simulink model "simple_streaming_txrx"  (Simulink 6.6)
settings: Solver=ode45  StartTime=0.0  StopTime=inf  RelTol=1e-3
InitFcn:
  | simple_streaming_init
StartFcn:
  | simple_streaming_init
undefined symbols (not defined in the file): dmf, gcbh, get, modConstellation_qam16, modConstellation_qam64, modConstellation_qpsk, rcosfir, symbolRomLen, txLSFR_initValues, txLSFR_polynomials, viqAvgLen, xlBlockLoadCallback, xlGetSimulinkPeriod
libraries: xbsIndex_r4 x506, commchan3 x2, commsink2 x1
(part 1 of 5)
settings Model: Creator=chunter  LastModifiedBy=chunter

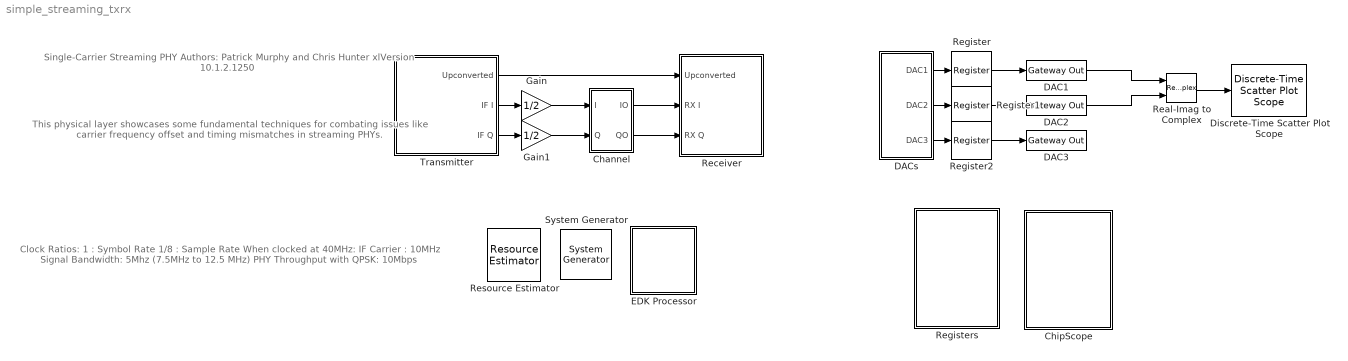
== system simple_streaming_txrx ==
  note: Single-Carrier Streaming PHY
      | Authors: Patrick Murphy and Chris Hunter
      | xlVersion 10.1.2.1250
  note: This physical layer showcases some fundamental
      | techniques for combating issues like carrier frequency
      | offset and timing mismatches in streaming PHYs.
  note: Clock Ratios:
      | 1 : Symbol Rate
      | 1/8 : Sample Rate
      |
      | When clocked at 40MHz:
      | IF Carrier : 10MHz
      | Signal Bandwidth: 5Mhz (7.5MHz to 12.5 MHz)
      | PHY Throughput with QPSK: 10Mbps
  " System Generator" : xbsIndex_r4/ System Generator  Tag=genX  SystemSampleTime=-1  xilinxfamily=virtex2p  part=xc2vp70  speed=-6  package=ff1517  synthesis_tool=XST  clock_wrapper=Clock Enables  directory=./netlist  testbench=off  simulink_period=1/8  sysclk_period=10  dcm_input_clock_period=100  incr_netlist=off  trim_vbits=Everywhere in SubSystem  dbl_ovrd=According to Block Masks  core_generation=According to Block Masks  run_coregen=off  deprecated_control=off  eval_field=0  block_type=sysgen
      settings: block_version=10.1.2
  Channel : Subsystem
  ChipScope : Subsystem
  DAC1 : xbsIndex_r4/Gateway Out  hdl_port=on  timing_constraint=None  locs_specified=off  LOCs={}  block_type=gatewayout
      settings: infoedit="Gateway out block.  Converts Xilinx fixed point inputs into ouputs of type Simulink integer, double, or fixed point.<P><P>Hardware notes:  In hardware these blocks become top level output ports or are discarded, depending on how they are configured."  xl_area=[0 0 0 0 14 0 0]  block_version=10.1
  DAC2 : xbsIndex_r4/Gateway Out  hdl_port=on  timing_constraint=None  locs_specified=off  LOCs={}  block_type=gatewayout
      settings: infoedit="Gateway out block.  Converts Xilinx fixed point inputs into ouputs of type Simulink integer, double, or fixed point.<P><P>Hardware notes:  In hardware these blocks become top level output ports or are discarded, depending on how they are configured."  xl_area=[0 0 0 0 14 0 0]  block_version=10.1
  DAC3 : xbsIndex_r4/Gateway Out  hdl_port=on  timing_constraint=None  locs_specified=off  LOCs={}  block_type=gatewayout
      settings: infoedit="Gateway out block.  Converts Xilinx fixed point inputs into ouputs of type Simulink integer, double, or fixed point.<P><P>Hardware notes:  In hardware these blocks become top level output ports or are discarded, depending on how they are configured."  xl_area=[0 0 0 0 14 0 0]  block_version=10.1
  DACs : Subsystem
  Discrete-Time Scatter Plot Scope : commsink2/Discrete-Time Scatter Plot Scope  Tag=ScatterPlot  SystemSampleTime=-1  sampPerSymb=1  offsetEye=0  numTraces=40  numNewFrames=10  LineMarkers=.  LineColors=b  fading=on  render=on  AxisGrid=on  xMin=-3.3  xMax=3.315  yMin=-3.3  yMax=3.315  inphaseLabel=In-phase Amplitude  quadratureLabel=Quadrature Amplitude  openScopeAtSimStart=on  FrameNumber=off  FigPos=get(0,'defaultfigureposition');  figTitle=Scatter Plot  numLinesMax=8  block_type_=scatter
  EDK Processor : Subsystem  LoadFcn=xlBlockLoadCallback(gcbh);  mask(Xilinx EDK Processor Block){mode=EDK pcore generation, xmp=, MemVisToProc=<qt bgcolor="#FFFFFF"><div><img src="C:\Xilinx\10.1\DSP_Tools\common\bin\..\..\sysgen\data\images\registerminus.gif"> &lt;&lt;cfoEnable&gt;&gt;<br> <img src="C:\Xilinx\10.1\DSP_Tools\common\bin\..\..\sysgen\data\images\parameters.gif"> Type : UFix_1_0<br> <img src="C:\Xilinx\10.1\DSP_Tools\common\bin\..\..\sysgen\data\images\parameters.gif"> Addr : 0x80000800<br></div><div><img src="C:\Xilinx\10.1\DSP_Tools\common\bin\..\..\sysgen\data\images\registerplus.gif"> &lt;&lt;cfoK&gt;&gt;<br></div><div><img src="C:\Xilinx\10.1\DSP_Tools\common\bin\..\..\sysgen\data\images\registerplus.gif"> &lt;&lt;cfoKI&gt;&gt;<br></div><div><img src="C:\Xilinx\10.1\DSP_Tools\common\bin\..\..\sysgen\data\images\registerplus.gif"> &lt;&lt;cfoKP&gt;&gt;<br></div><div><img src="C:\Xilinx\10.1\DSP_Tools\common\bin\..\..\sysgen\data\images\registerplus.gif"> &lt;&lt;cfoReset&gt;&gt;<br></div><div><img src="C:\Xilinx\10.1\DSP_Tools\common\bin\..\..\sysgen\data\images\registerplus.gif"> &lt;&lt;dac1Sel&gt;&gt;<br></div><div><img src="C:\Xilinx\10.1\DSP_Tools\common\bin\..\..\sysgen\data\images\registerplus.gif"> &lt;&lt;dac2Sel&gt;&gt;<br></div><div><img src="C:\Xilinx\10.1\DSP_Tools\common\bin\..\..\sysgen\data\images\registerplus.gif"> &lt;&lt;dac3Sel&gt;&gt;<br></div><div><img src="C:\Xilinx\10.1\DSP_Tools\common\bin\..\..\sysgen\data\images\registerplus.gif"> &lt;&lt;downConv&gt;&gt;<br></div><div><img src="C:\Xilinx\10.1\DSP_Tools\common\bin\..\..\sysgen\data\images\registerplus.gif"> &lt;&lt;initialDelay&gt;&gt;<br></div><div><img src="C:\Xilinx\10.1\DSP_Tools\common\bin\..\..\sysgen\data\images\registerminus.gif"> &lt;&lt;otrBenefit&gt;&gt;<br> <img src="C:\Xilinx\10.1\DSP_Tools\common\bin\..\..\sysgen\data\images\parameters.gif"> Type : UFix_32_0<br> <img src="C:\Xilinx\10.1\DSP_Tools\common\bin\..\..\sysgen\data\images\parameters.gif"> Addr : 0x80000828<br></div><div><img src="C:\Xilinx\10.1\DSP_Tools\common\bin\..\..\sysgen\data\images\registerplus.gif"> &lt;&lt;otrCost&gt;&gt;<br></div><div><img src="C:\Xilinx\10.1\DSP_Tools\common\bin\..\..\sysgen\data\images\registerplus.gif"> &lt;&lt;rxInputSel&gt;&gt;<br></div><div><img src="C:\Xilinx\10.1\DSP_Tools\common\bin\..\..\sysgen\data\images\registerplus.gif"> &lt;&lt;timingK&gt;&gt;<br></div><div><img src="C:\Xilinx\10.1\DSP_Tools\common\bin\..\..\sysgen\data\images\registerplus.gif"> &lt;&lt;timingKI&gt;&gt;<br></div><div><img src="C:\Xilinx\10.1\DSP_Tools\common\bin\..\..\sysgen\data\images\registerplus.gif"> &lt;&lt;timingKP&gt;&gt;<br></div><div><img src="C:\Xilinx\10.1\DSP_Tools\common\bin\..\..\sysgen\data\images\registerplus.gif"> &lt;&lt;timingReset&gt;&gt;<br></div><div><img src="C:\Xilinx\10.1\DSP_Tools\common\bin\..\..\sysgen\data\images\registerplus.gif"> &lt;&lt;txModSel&gt;&gt;<br></div><div><img src="C:\Xilinx\10.1\DSP_Tools\common\bin\..\..\sysgen\data\images\registerminus.gif"> &lt;&lt;upConv&gt;&gt;<br> <img src="C:\Xilinx\10.1\DSP_Tools\common\bin\..\..\sysgen\data\images\parameters.gif"> Type : UFix_32_0<br> <img src="C:\Xilinx\10.1\DSP_Tools\common\bin\..\..\sysgen\data\images\parameters.gif"> Addr : 0x80000848<br></div><div><img src="C:\Xilinx\10.1\DSP_Tools\common\bin\..\..\sysgen\data\images\registerminus.gif"> &lt;&lt;otr&gt;&gt;<br> <img src="C:\Xilinx\10.1\DSP_Tools\common\bin\..\..\sysgen\data\images\parameters.gif"> Type : UFix_32_0<br> <img src="C:\Xilinx\10.1\DSP_Tools\common\bin\..\..\sysgen\data\images\parameters.gif"> Addr : 0x80000850<br></div><div><img src="C:\Xilinx\10.1\DSP_Tools\common\bin\..\..\sysgen\data\images\registerminus.gif"> &lt;&lt;rssi&gt;&gt;<br> <img src="C:\Xilinx\10.1\DSP_Tools\common\bin\..\..\sysgen\data\images\parameters.gif"> Type : UFix_32_0<br> <img src="C:\Xilinx\10.1\DSP_Tools\common\bin\..\..\sysgen\data\images\parameters.gif"> Addr : 0x80000854<br></div><div><img src="C:\Xilinx\10.1\DSP_Tools\common\bin\..\..\sysgen\data\images\registerplus.gif"> &lt;&lt;viq&gt;&gt;<br></div><div><img src="C:\Xilinx\10.1\DSP_Tools\common\bin\..\..\sysgen\data\images\registerplus.gif"> &lt;&lt;viqReset&gt;&gt;<br></div></qt>, AvailableMemories=<empty>, portInterfaceTable={'exposed'=>[],'portdir'=>[],'portname'=>[],'shortname'=>[]}, bus_type_sgadvanced=, bus_type=PLB, baseaddr=0x80000000, baseaddr_lock_sgadvanced=, baseaddr_lock=off, dual_clock_sgadvanced=, dual_clock=off, ucf_file=, inheritDeviceType_sgadvanced=, inheritDeviceType=off, clock_name=plb, internalPortList={}, resetPolarity=0, memxtable={'mlist'=>['simple_streaming_txrx/Registers/From Register16','simple_streaming_txrx/Registers/From Register12','simple_streaming_txrx/Registers/From Register13','simple_streaming_txrx/Registers/From Register14','simple_streaming_txrx/Registers/From Register11','simple_streaming_txrx/Registers/From Register','simple_streaming_txrx/Registers/From Register1','simple_streaming_txrx/Registers/From Register4','simple_streaming_txrx/Registers/From Register5','simple_streaming_txrx/Registers/From Register15','simple_streaming_txrx/Registers/From Register17','simple_streaming_txrx/Registers/From Register18','simple_streaming_txrx/Registers/From Register6','simple_streaming_txrx/Registers/From Register7','simple_streaming_txrx/Registers/From Register9','simple_streaming_txrx/Registers/From Register8','simple_streaming_txrx/Registers/From Register10','simple_streaming_txrx/Registers/From Register2','simple_streaming_txrx/Registers/From Register3','simple_streaming_txrx/Registers/To Register2','simple_streaming_txrx/Registers/To Register1','simple_streaming_txrx/Registers/To Register','simple_streaming_txrx/Registers/From Register19'],'mlname'=>['\'cfoEnable\'','\'cfoK\'','\'cfoKI\'','\'cfoKP\'','\'cfoReset\'','\'dac1Sel\'','\'dac2Sel\'','\'dac3Sel\'','\'downConv\'','\'initialDelay\'','\'otrBenefit\'','\'otrCost\'','\'rxInputSel\'','\'timingK\'','\'timingKI\'','\'timingKP\'','\'timingReset\'','\'txModSel\'','\'upConv\'','\'otr\'','\'rssi\'','\'viq\'','\'viqReset\''],'mlstate'=>[1.0000000000000000,0.00000000000000000,0.00000000000000000,0.00000000000000000,0.00000000000000000,0.00000000000000000,0.00000000000000000,0.00000000000000000,0.00000000000000000,0.00000000000000000,1.0000000000000000,0.00000000000000000,0.00000000000000000,0.00000000000000000,0.00000000000000000,0.00000000000000000,0.00000000000000000,0.00000000000000000,1.0000000000000000,1.0000000000000000,1.0000000000000000,0.00000000000000000,0.00000000000000000]}, procinfo={'xmliface'=>'Xilinx//microblaze//iface.xml'}, fslifaceports=[0,0], memmapdirty=off, blockname=, xpsintstyle=default, proc=, has_advanced_control=0, sggui_pos=20,20,383,441, block_type=edkprocessor, block_version=2.4, sg_icon_stat=62,64,-1,-1,white,blue,0,07734,right, sg_mask_display=|, sg_list_contents={'table'=>{'AvailableMemories'=>'popup(<empty>)','userSelections'=>{'AvailableMemories'=>'<empty>'}}}, sg_blockgui_xml=}
      mask sg_mask_display=|
      | fprintf('','COMMENT: begin icon graphics');
      | patch([0 62 62 0 ],[0 0 64 64 ],[0.77 0.82 0.91]);
      | patch([14 4 19 4 14 30 34 38 56 42 29 19 33 19 29 42 56 38 34 30 14 ],[8 18 33 48 58 58 54 58 58 44 57 47 33 19 9 22 8 8 12 8 8 ],[0.98 0.96 0.92]);
      | plot([0 62 62 0 0 ],[0 0 64 64 0 ]);
      | fprintf('','COMMENT: end icon graphics');
      | fprintf('','COMMENT: begin icon text');
      | fprintf('','COMMENT: end icon text');
      mask prompts: mode "Configure Processor for"; xmp "EDK Project"; MemVisToProc ""; AvailableMemories "Available Memories"; portInterfaceTable ""; bus_type_sgadvanced ""; bus_type "Bus Type"; baseaddr "Base Address"; baseaddr_lock_sgadvanced ""; baseaddr_lock "Lock"; dual_clock_sgadvanced ""; dual_clock "Dual Clocks"; ucf_file "Constraint file"; inheritDeviceType_sgadvanced ""; inheritDeviceType "Inherit Device Type"; clock_name ""; internalPortList ""; resetPolarity ""; memxtable ""; procinfo ""; fslifaceports ""; memmapdirty ""; blockname ""; xpsintstyle ""; proc ""; has_advanced_control ""; sggui_pos ""; block_type ""; block_version ""; sg_icon_stat ""; sg_mask_display ""; sg_list_contents ""; sg_blockgui_xml ""
      mask help: Xilinx EDK Processor
      mask init:
      | try
      |   tmp_gcb = gcb;
      |   tmp_gcbh = gcbh;
      |   if (strcmp('SysGenIndex',get_param(bdroot(tmp_gcbh),'tag')) && ~isempty(regexp(bdroot(tmp_gcb), '^xbs', 'once')))
      |     return;
      |   end;
      |   xlMungeMaskParams;
      |   serialized_declarations = '{}';
      |   xledkprocessor_init();
      |   ptable_ = xlblockprep(get_param(tmp_gcb, 'MaskWSVariables'));
      | catch
      |   global dbgsysgen;
      |   if(~isempty(dbgsysgen) && dbgsysgen)
      |     e = regexprep(lasterr, '\n', '\nError: ');
      |     disp(['Error: While running MaskInit code on block ' tmp_gcb ': ' e]);
      |     error(e);
      |   end
      | end
      settings: CopyFcn=xlProcBlockCopyCallback(gcbh);xlBlockMoveCallback(gcbh);  DeleteFcn=xlDestroyGui(gcbh);  ModelCloseFcn=xlDestroyGui(gcbh);  PreSaveFcn=xlBlockPreSaveCallback(gcbh);  PostSaveFcn=xlBlockPostSaveCallback(gcbh);  DestroyFcn=xlDestroyGui(gcbh);  OpenFcn=bh=gcbh;xlProcBlockCallbacks('populatesharedmemorylistbox',bh);xlOpenGui(bh, 'edkprocessor_gui.xml', @xlProcBlockEnablement, @xlProcBlockAction)  CloseFcn=xlDestroyGui(gcbh);  MoveFcn=xlBlockMoveCallback(gcbh);
      mask Help: eval('');xlDoc('-book','sysgen','-topic','EDK_Processor');
      mask StyleString: popup(EDK pcore generation|HDL netlisting),edit,edit,popup(<empty>),edit,edit,popup(PLB|FSL),edit,edit,checkbox,edit,checkbox,edit,edit,checkbox,edit,edit,edit,edit,edit,edit,edit,edit,edit,edit,edit,edit,edit,edit,edit,edit,edit,edit
      mask Display:
      | fprintf('','COMMENT: begin icon graphics');
      | patch([0 62 62 0 ],[0 0 64 64 ],[0.77 0.82 0.91]);
      | patch([14 4 19 4 14 30 34 38 56 42 29 19 33 19 29 42 56 38 34 30 14 ],[8 18 33 48 58 58 54 58 58 44 57 47 33 19 9 22 8 8 12 8 8 ],[0.98 0.96 0.92]);
      | plot([0 62 62 0 0 ],[0 0 64 64 0 ]);
      | fprintf('','COMMENT: end icon graphics');
      | fprintf('','COMMENT: begin icon text');
      | disp('MicroBlaze');
      | 
      | fprintf('','COMMENT: end icon text');
  Gain : Gain  Gain=1/2
  Gain1 : Gain  Gain=1/2
  Real-Imag to Complex : RealImagToComplex
  Receiver : Subsystem
  Register : xbsIndex_r4/Register  init=0  rst=off  en=off  dbl_ovrd=off  block_type=register
      settings: xl_area=[7 14 0 0 0 0 0]  block_version=10.1
  Register1 : xbsIndex_r4/Register  init=0  rst=off  en=off  dbl_ovrd=off  block_type=register
      settings: xl_area=[7 14 0 0 0 0 0]  block_version=10.1
  Register2 : xbsIndex_r4/Register  init=0  rst=off  en=off  dbl_ovrd=off  block_type=register
      settings: xl_area=[7 14 0 0 0 0 0]  block_version=10.1
  Registers : Subsystem
  Resource Estimator : xbsIndex_r4/Resource Estimator  Tag=resEstTag  Slices=3401  FFs=3180  BRAMs=6  LUTs=4413  IOBs=244  EBMs=75  TBUFs=0  xl_use_estimator_area=off  est_options=Estimate  block_type=resource_estimator
      settings: AttributesFormatString=Resource\nEstimator  block_version=10.1.2
  Transmitter : Subsystem
  wires:
  DACs/1(DAC1) -> Register/1
  DACs/2(DAC2) -> Register1/1
  DACs/3(DAC3) -> Register2/1
  Transmitter/1(Upconverted) -> Receiver/1(Upconverted)
  Gain/1 -> Channel/1(I)
  Gain1/1 -> Channel/2(Q)
  Register/1 -> DAC1/1
  Register1/1 -> DAC2/1
  Register2/1 -> DAC3/1
  Transmitter/2(IF I) -> Gain/1
  Transmitter/3(IF Q) -> Gain1/1
  Real-Imag to Complex/1 -> Discrete-Time Scatter Plot Scope/1
  DAC1/1 -> Real-Imag to Complex/1
  DAC2/1 -> Real-Imag to Complex/2
  Channel/1(IO) -> Receiver/2(RX I)
  Channel/2(QO) -> Receiver/3(RX Q)

== system simple_streaming_txrx/Channel ==
  I : Inport
  Q : Inport  Port=2
  AWGN Channel : commchan3/AWGN Channel  SystemSampleTime=-1  seed=67  noiseMode="Signal to noise ratio  (Eb/No)"  EbNodB=40  EsNodB=10  SNRdB=10  bitsPerSym=1  Ps=1  Tsym=1  variance=1
  AWGN Channel1 : commchan3/AWGN Channel  SystemSampleTime=-1  seed=30  noiseMode="Signal to noise ratio  (Eb/No)"  EbNodB=40  EsNodB=10  SNRdB=10  bitsPerSym=1  Ps=1  Tsym=1  variance=1
  IO : Outport
  QO : Outport  Port=2
  wires:
  I/1 -> AWGN Channel/1
  AWGN Channel/1 -> IO/1
  Q/1 -> AWGN Channel1/1
  AWGN Channel1/1 -> QO/1

== system simple_streaming_txrx/ChipScope ==
  ChipScope : xbsIndex_r4/ChipScope  num_trig_ports=1  current_port=0  show_trig_port=0  match_units=1  match_type=Basic  data_is_trigger=off  num_data_ports=13  data_depth=8192  SRL16s=on  match_type_t0=1  match_type_t1=1  match_type_t2=1  match_type_t3=1  match_type_t4=1  match_type_t5=1  match_type_t6=1  match_type_t7=1  match_type_t8=1  match_type_t9=1  match_type_t10=1  match_type_t11=1  match_type_t12=1  match_type_t13=1  match_type_t14=1  match_type_t15=1  match_units_t0=1  match_units_t1=1  match_units_t2=1  match_units_t3=1  match_units_t4=1  match_units_t5=1  match_units_t6=1  match_units_t7=1  match_units_t8=1  match_units_t9=1  match_units_t10=1  match_units_t11=1  match_units_t12=1  match_units_t13=1  match_units_t14=1  match_units_t15=1  dbl_ovrd=0  block_type=chipscope
      settings: infoedit="Enables run-time debugging and verification of signals by inserting ChipScope Pro ICON and ILA cores.<br><br>  Restrictions: <br>Only one ChipScope core can be instantiated in a System Generator design.This block cannot be used at the same time as JTAG hardware co-simulation.A design or subsystem containing a ChipScope block must have at least one output port."  block_version=10.1
  chipscope_trigger : xbsIndex_r4/Gateway In  arith_type=Unsigned  n_bits=1  bin_pt=0  quantization="Round  (unbiased: +/- Inf)"  overflow=Saturate  period=1  dbl_ovrd=off  timing_constraint=None  locs_specified=off  LOCs={}  block_type=gatewayin
      settings: infoedit="Gateway in block.  Converts inputs of type Simulink integer, double and fixed point to  Xilinx fixed point type.<P><P>Hardware notes:  In hardware these blocks become top level input ports."  xl_area=[0 0 0 0 1 0 0]  block_version=10.1
  wires:
  chipscope_trigger/1 -> ChipScope/1
  [Symbols_Tx_I] -> ChipScope/2  "Symbols_Tx_I"
  [Symbols_Tx_Q] -> ChipScope/3  "Symbols_Tx_Q"
  [Symbols_Filt_I] -> ChipScope/4  "Symbols_Filt_I"
  [Symbols_Filt_Q] -> ChipScope/5  "Symbols_Filt_Q"
  [Upconverted] -> ChipScope/6  "Upconverted"
  [PHASEERROR] -> ChipScope/7  "PHASEERROR"
  [CFOINC] -> ChipScope/8  "CFOINC"
  [TED] -> ChipScope/9  "TED"
  [TEDFILT] -> ChipScope/10  "TEDFILT"
  [dly] -> ChipScope/11  "dly"
  [Symbols_Rx_I] -> ChipScope/12  "Symbols_Rx_I"
  [Symbols_Rx_Q] -> ChipScope/13  "Symbols_Rx_Q"
  [RXINPUT] -> ChipScope/14  "RXINPUT"

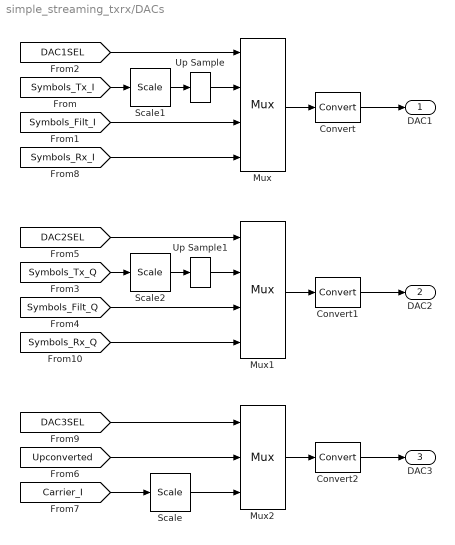
== system simple_streaming_txrx/DACs ==
  Convert : xbsIndex_r4/Convert  arith_type="Signed  (2's comp)"  n_bits=14  bin_pt=13  quantization=Truncate  overflow=Wrap  latency=0  dbl_ovrd=off  pipeline=off  block_type=convert
      settings: xl_area=[0 0 0 0 0 0 0]  block_version=10.1
  Convert1 : xbsIndex_r4/Convert  arith_type="Signed  (2's comp)"  n_bits=14  bin_pt=13  quantization=Truncate  overflow=Wrap  latency=0  dbl_ovrd=off  pipeline=off  block_type=convert
      settings: xl_area=[0 0 0 0 0 0 0]  block_version=10.1
  Convert2 : xbsIndex_r4/Convert  arith_type="Signed  (2's comp)"  n_bits=14  bin_pt=13  quantization=Truncate  overflow=Wrap  latency=0  dbl_ovrd=off  pipeline=off  block_type=convert
      settings: xl_area=[0 0 0 0 0 0 0]  block_version=10.1
  Mux : xbsIndex_r4/Mux  inputs=3  en=off  latency=0  precision=Full  arith_type=Unsigned  n_bits=16  bin_pt=14  quantization=Truncate  overflow=Wrap  dbl_ovrd=off  block_type=mux
      settings: xl_area=[17 0 0 34 0 0 0]  block_version=10.1
  Mux1 : xbsIndex_r4/Mux  inputs=3  en=off  latency=0  precision=Full  arith_type=Unsigned  n_bits=16  bin_pt=14  quantization=Truncate  overflow=Wrap  dbl_ovrd=off  block_type=mux
      settings: xl_area=[17 0 0 34 0 0 0]  block_version=10.1
  Mux2 : xbsIndex_r4/Mux  inputs=2  en=off  latency=0  precision=Full  arith_type=Unsigned  n_bits=16  bin_pt=14  quantization=Truncate  overflow=Wrap  dbl_ovrd=off  block_type=mux
      settings: xl_area=[9 0 0 17 0 0 0]  block_version=10.1
  Scale : xbsIndex_r4/Scale  scale_factor=-1  dbl_ovrd=off  block_type=scale
      settings: infoedit=Scales input by a power of two by adjusting the binary point position.<P><P>Hardware notes: In hardware this block costs nothing.  block_version=10.1
  Scale1 : xbsIndex_r4/Scale  scale_factor=-1  dbl_ovrd=off  block_type=scale
      settings: infoedit=Scales input by a power of two by adjusting the binary point position.<P><P>Hardware notes: In hardware this block costs nothing.  block_version=10.1
  Scale2 : xbsIndex_r4/Scale  scale_factor=-1  dbl_ovrd=off  block_type=scale
      settings: infoedit=Scales input by a power of two by adjusting the binary point position.<P><P>Hardware notes: In hardware this block costs nothing.  block_version=10.1
  Up Sample : xbsIndex_r4/Up Sample  sample_ratio=8  copy_samples=on  dbl_ovrd=off  block_type=usamp
      settings: infoedit="Up samples input data.  Inserted values  can be zeros or copies of the most recent input sample.<P><P>Hardware notes: No hardware is needed if inserted values are copies of the input sample; otherwise, a mux and single bit flip-flop are used."  xl_area=[0 0 0 0 0 0 0]  block_version=10.1
  Up Sample1 : xbsIndex_r4/Up Sample  sample_ratio=8  copy_samples=on  dbl_ovrd=off  block_type=usamp
      settings: infoedit="Up samples input data.  Inserted values  can be zeros or copies of the most recent input sample.<P><P>Hardware notes: No hardware is needed if inserted values are copies of the input sample; otherwise, a mux and single bit flip-flop are used."  xl_area=[0 0 0 0 0 0 0]  block_version=10.1
  DAC1 : Outport
  DAC2 : Outport  Port=2
  DAC3 : Outport  Port=3
  wires:
  [Symbols_Tx_I] -> Scale1/1
  [Symbols_Filt_I] -> Mux/3
  [DAC1SEL] -> Mux/1
  [Symbols_Tx_Q] -> Scale2/1
  [Symbols_Filt_Q] -> Mux1/3
  [DAC2SEL] -> Mux1/1
  Mux/1 -> Convert/1
  Mux1/1 -> Convert1/1
  Mux2/1 -> Convert2/1
  [Upconverted] -> Mux2/2
  [Carrier_I] -> Scale/1
  [DAC3SEL] -> Mux2/1
  Convert/1 -> DAC1/1
  Convert1/1 -> DAC2/1
  Convert2/1 -> DAC3/1
  Up Sample/1 -> Mux/2
  Up Sample1/1 -> Mux1/2
  [Symbols_Rx_I] -> Mux/4
  [Symbols_Rx_Q] -> Mux1/4
  Scale/1 -> Mux2/3
  Scale1/1 -> Up Sample/1
  Scale2/1 -> Up Sample1/1
